simulink model "thermostat_schedule"  (Simulink 7.6)
settings: Solver=ode45  StartTime=0.0  StopTime=24  RelTol=1e-3
settings Model: Creator=jm3gonza  LastModifiedBy=jm3gonza

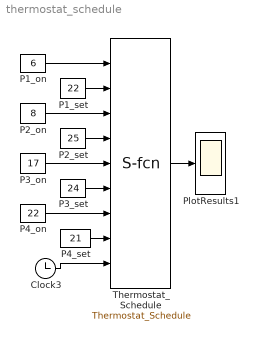
== system thermostat_schedule ==
  Clock3 : Clock
      settings: Decimation=1000
  P1_on : Constant  Value=6
  P1_set : Constant  Value=22
  P2_on : Constant  Value=8
  P2_set : Constant  Value=25
  P3_on : Constant  Value=17
  P3_set : Constant  Value=24
  P4_on : Constant  Value=22
  P4_set : Constant  Value=21
  PlotResults1 : Scope
      settings: TimeRange=24  YMin=15  YMax=18  SaveName=a  DataFormat=Array
  Thermostat_Schedule : M-S-Function  FunctionName=Thermostat_Schedule
      mask Display: port_label('output', 1, 'ON/OFF')
  wires:
  P1_on/1 -> Thermostat_Schedule/1
  P1_set/1 -> Thermostat_Schedule/2
  P2_on/1 -> Thermostat_Schedule/3
  P2_set/1 -> Thermostat_Schedule/4
  P3_on/1 -> Thermostat_Schedule/5
  P3_set/1 -> Thermostat_Schedule/6
  P4_on/1 -> Thermostat_Schedule/7
  P4_set/1 -> Thermostat_Schedule/8
  Clock3/1 -> Thermostat_Schedule/9
  Thermostat_Schedule/1 -> PlotResults1/1
